simulink library "csc_ekf_nonlinear_filter_mtv_lib"  (R2014b)
settings: Solver=ode45  SolverMode=SingleTasking  StartTime=0.0  StopTime=10.0  RelTol=1e-3
undefined symbols (not defined in the file or in its folder): fcv_initializing
libraries: simulink x2, util_info_lib x1, csc_sqt_sequential_trigger_mtv_lib x1, csc_tup_time_update_lib x1, csu_mkf_multiplicative_update_mtv_lib x1
settings Model: ExtModeAutoUpdateStatusClock=off  Creator=escrane  LastModifiedBy=mstewart

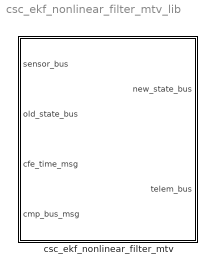
== system csc_ekf_nonlinear_filter_mtv_lib ==
  csc_ekf_nonlinear_filter_mtv : Subsystem

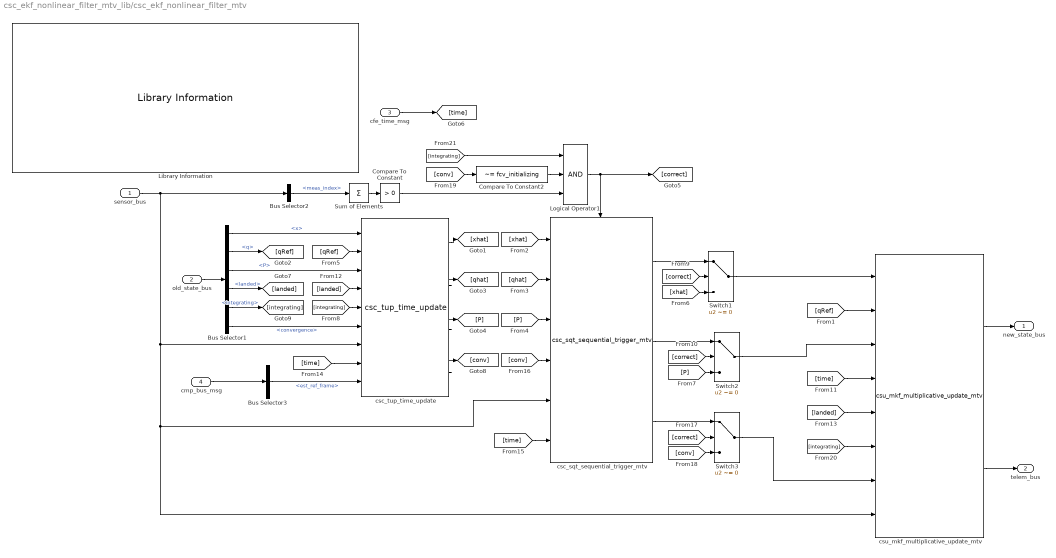
== system csc_ekf_nonlinear_filter_mtv_lib/csc_ekf_nonlinear_filter_mtv ==
  sensor_bus : Inport
  old_state_bus : Inport  Port=2
  cfe_time_msg : Inport  Port=3
  cmp_bus_msg : Inport  Port=4
  Bus Selector1 : BusSelector  OutputSignals=x,q,P,landed,integrating,convergence
  Bus Selector2 : BusSelector  OutputSignals=meas_index
  Bus Selector3 : BusSelector  OutputSignals=est_ref_frame
  Compare To Constant : simulink/Logic and Bit Operations/Compare To Constant  relop=>  const=0  OutDataTypeStr=uint8  ZeroCross=off
  Compare To Constant2 : simulink/Logic and Bit Operations/Compare To Constant  relop=~=  const=fcv_initializing  OutDataTypeStr=boolean
  Library Information : util_info_lib/Library Information  owner='NONE'
  Logical Operator1 : Logic  Inputs=3  AllPortsSameDT=off  OutDataTypeStr=boolean
  Sum of Elements : Sum  Inputs=+
  Switch1 : Switch  Criteria=u2 ~= 0  Threshold=0.5  InputSameDT=on
  Switch2 : Switch  Criteria=u2 ~= 0  Threshold=0.5  InputSameDT=on
  Switch3 : Switch  Criteria=u2 ~= 0  Threshold=0.5  InputSameDT=on
  csc_sqt_sequential_trigger_mtv : csc_sqt_sequential_trigger_mtv_lib/csc_sqt_sequential_trigger_mtv
  csc_tup_time_update : csc_tup_time_update_lib/csc_tup_time_update
  csu_mkf_multiplicative_update_mtv : csu_mkf_multiplicative_update_mtv_lib/csu_mkf_multiplicative_update_mtv
  new_state_bus : Outport
  telem_bus : Outport  Port=2
  wires:
  Switch2/1 -> csu_mkf_multiplicative_update_mtv/3
  [integrating] -> Logical Operator1/1
  [integrating] -> csu_mkf_multiplicative_update_mtv/6
  Bus Selector1/6 -> csc_tup_time_update/6  "<convergence>"
  Bus Selector1/5 -> [integrating]  "<integrating>"
  [integrating] -> csc_tup_time_update/5
  Compare To Constant/1 -> Logical Operator1/3
  Compare To Constant2/1 -> Logical Operator1/2
  [conv] -> Compare To Constant2/1
  Logical Operator1/1 -> [correct], csc_sqt_sequential_trigger_mtv/Enable
  csc_sqt_sequential_trigger_mtv/3 -> Switch3/1
  [conv] -> Switch3/3
  [correct] -> Switch3/2
  [conv] -> csc_sqt_sequential_trigger_mtv/4
  csc_tup_time_update/4 -> [conv]
  cfe_time_msg/1 -> [time]
  [landed] -> csu_mkf_multiplicative_update_mtv/5
  [landed] -> csc_tup_time_update/4
  Bus Selector1/4 -> [landed]  "<landed>"
  cmp_bus_msg/1 -> Bus Selector3/1
  Bus Selector3/1 -> csc_tup_time_update/9  "<est_ref_frame>"
  [time] -> csc_tup_time_update/8
  [qRef] -> csc_tup_time_update/2
  Bus Selector1/3 -> csc_tup_time_update/3  "<P>"
  sensor_bus/1 -> Bus Selector2/1, csc_tup_time_update/7, csc_sqt_sequential_trigger_mtv/5, csu_mkf_multiplicative_update_mtv/8
  Bus Selector1/1 -> csc_tup_time_update/1  "<x>"
  old_state_bus/1 -> Bus Selector1/1
  Bus Selector1/2 -> [qRef]  "<q>"
  [qRef] -> csu_mkf_multiplicative_update_mtv/2
  csc_tup_time_update/1 -> [xhat]
  [xhat] -> csc_sqt_sequential_trigger_mtv/1
  csc_tup_time_update/2 -> [qhat]
  [qhat] -> csc_sqt_sequential_trigger_mtv/2
  csc_tup_time_update/3 -> [P]
  [P] -> csc_sqt_sequential_trigger_mtv/3
  csc_sqt_sequential_trigger_mtv/1 -> Switch1/1
  [xhat] -> Switch1/3
  csc_sqt_sequential_trigger_mtv/2 -> Switch2/1
  Bus Selector2/1 -> Sum of Elements/1  "<meas_index>"
  Sum of Elements/1 -> Compare To Constant/1
  [correct] -> Switch1/2
  [P] -> Switch2/3
  [correct] -> Switch2/2
  Switch1/1 -> csu_mkf_multiplicative_update_mtv/1
  [time] -> csc_sqt_sequential_trigger_mtv/6
  [time] -> csu_mkf_multiplicative_update_mtv/4
  Switch3/1 -> csu_mkf_multiplicative_update_mtv/7
  csu_mkf_multiplicative_update_mtv/1 -> new_state_bus/1
  csu_mkf_multiplicative_update_mtv/2 -> telem_bus/1
